simulink model "a23_parallel"  (R2014a)
settings: Solver=ode45  StartTime=0.0  StopTime=10.0  RelTol=1e-3
settings Model: Creator=s65556  LastModifiedBy=s65556

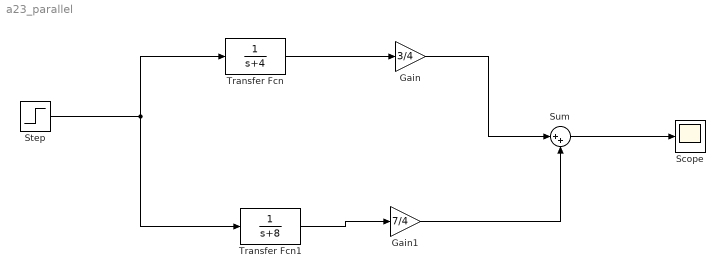
== system a23_parallel ==
  Gain : Gain  Gain=3/4
  Gain1 : Gain  Gain=7/4
  Scope : Scope
  Step : Step  SampleTime=0
  Sum : Sum  Inputs=|++
  Transfer Fcn : TransferFcn  Denominator=[1 4]
  Transfer Fcn1 : TransferFcn  Denominator=[1 8]
  wires:
  Transfer Fcn/1 -> Gain/1
  Gain/1 -> Sum/1
  Step/1 -> Transfer Fcn1/1, Transfer Fcn/1
  Transfer Fcn1/1 -> Gain1/1
  Gain1/1 -> Sum/2
  Sum/1 -> Scope/1
